simulink model "ques3"  (R2021a)
settings: Solver=VariableStepAuto  StartTime=0.0  StopTime=0.1  RelTol=1e-3
settings Model: Creator=AVM  LastModifiedBy=AVM

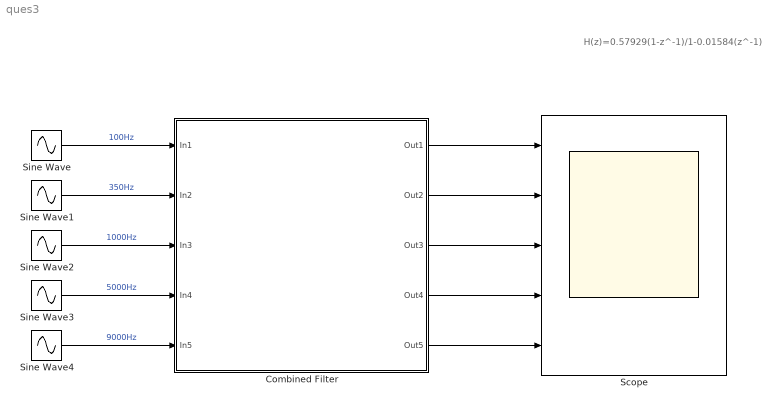
== system ques3 ==
  note: H(z)=0.57929(1-z^-1)/1-0.01584(z^-1)
  " Combined Filter" : Subsystem
  Scope : Scope  NumInputPorts=5
  Sine Wave : Sin  Frequency=2*pi*100  SampleTime=0
  Sine Wave1 : Sin  Frequency=2*pi*350  SampleTime=0
  Sine Wave2 : Sin  Frequency=2*pi*1000  SampleTime=0
  Sine Wave3 : Sin  Frequency=2*pi*5000  SampleTime=0
  Sine Wave4 : Sin  Frequency=2*pi*9000  SampleTime=0
  wires:
  Sine Wave/1 -> " Combined Filter"/1(In1)  "100Hz"
  Sine Wave1/1 -> " Combined Filter"/2(In2)  "350Hz"
  Sine Wave2/1 -> " Combined Filter"/3(In3)  "1000Hz"
  Sine Wave3/1 -> " Combined Filter"/4(In4)  "5000Hz"
  Sine Wave4/1 -> " Combined Filter"/5(In5)  "9000Hz"
  " Combined Filter"/1(Out1) -> Scope/1
  " Combined Filter"/2(Out2) -> Scope/2
  " Combined Filter"/3(Out3) -> Scope/3
  " Combined Filter"/4(Out4) -> Scope/4
  " Combined Filter"/5(Out5) -> Scope/5

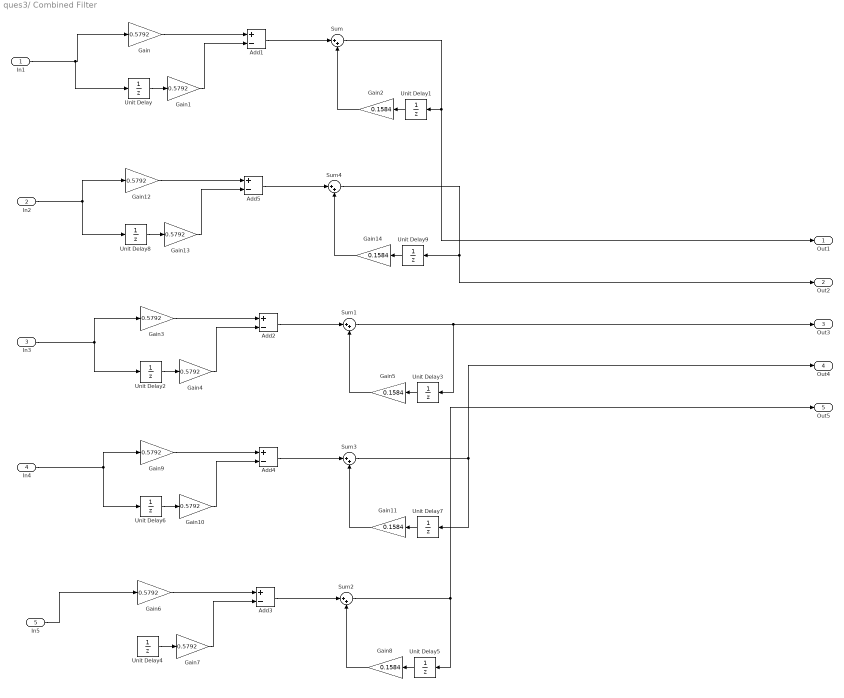
== system ques3/ Combined Filter ==
  In1 : Inport
  In2 : Inport  Port=2
  In3 : Inport  Port=3
  In4 : Inport  Port=4
  In5 : Inport  Port=5
  Add{1..5} (5 alike) : Sum  Inputs=+-
  Gain{,1,3..4,6..7,9..10,12..13} (10 alike) : Gain  Gain=0.5792
  Gain{2,5,8,11,14} (5 alike) : Gain  Gain=0.1584
  Sum{,1..4} (5 alike) : Sum  Inputs=|++
  Unit Delay{,1..9} (10 alike) : UnitDelay  SampleTime=-1  HasFrameUpgradeWarning=on
  Out1 : Outport
  Out2 : Outport  Port=2
  Out3 : Outport  Port=3
  Out4 : Outport  Port=4
  Out5 : Outport  Port=5
  wires:
  Unit Delay5/1 -> Gain8/1
  Gain3/1 -> Add2/1
  Sum2/1 -> Out5/1, Unit Delay5/1
  Gain12/1 -> Add5/1
  In4/1 -> Unit Delay6/1, Gain9/1
  Unit Delay1/1 -> Gain2/1
  Gain1/1 -> Add1/2
  In1/1 -> Unit Delay/1, Gain/1
  Gain9/1 -> Add4/1
  In2/1 -> Unit Delay8/1, Gain12/1
  Add3/1 -> Sum2/1
  Unit Delay4/1 -> Gain7/1
  Sum3/1 -> Out4/1, Unit Delay7/1
  Gain11/1 -> Sum3/2
  Sum1/1 -> Out3/1, Unit Delay3/1
  Sum/1 -> Out1/1, Unit Delay1/1
  Gain5/1 -> Sum1/2
  Sum4/1 -> Out2/1, Unit Delay9/1
  Unit Delay/1 -> Gain1/1
  Gain/1 -> Add1/1
  Unit Delay2/1 -> Gain4/1
  Add1/1 -> Sum/1
  Gain14/1 -> Sum4/2
  ? -> Unit Delay4/1
  Gain2/1 -> Sum/2
  Gain8/1 -> Sum2/2
  Unit Delay8/1 -> Gain13/1
  Unit Delay7/1 -> Gain11/1
  Add4/1 -> Sum3/1
  Unit Delay6/1 -> Gain10/1
  In3/1 -> Unit Delay2/1, Gain3/1
  Add5/1 -> Sum4/1
  Gain10/1 -> Add4/2
  Gain7/1 -> Add3/2
  Add2/1 -> Sum1/1
  Unit Delay9/1 -> Gain14/1
  Gain13/1 -> Add5/2
  Unit Delay3/1 -> Gain5/1
  Gain4/1 -> Add2/2
  Gain6/1 -> Add3/1
  In5/1 -> Gain6/1
